simulink model "model_sinWave_1D"  (R2016b)
settings: Solver=FixedStepAuto  StartTime=0.0  StopTime=160  FixedStep=0.001  RelTol=1e-3  EnableMultiTasking=on
InitFcn:
  | initCallback_model1D
values from neighbouring files (symbols this model uses):
  f_sine = fArr(k)    [simulationMessung.m]
undefined symbols (not defined in the file or in its folder): C_phi, C_psi, g, I_GO, I_RM, l_AB, l_AC, m_K, m_R, phi_0, phi__d_0, phi_off, psi_0, psi__d_0, T_M_e, T_M_m
settings Model: Creator=ich  LastModifiedBy=ich
settings SolverCC: AutoInsertRateTranBlk=on
settings OptimizationCC: LifeSpan=inf
settings DebuggingCC: AlgebraicLoopMsg=none  SFUnexpectedBacktrackingDiag=warning  SFNoUnconditionalDefaultTransitionDiag=warning  SFExecutionAtInitializationDiag=none
settings GRTTargetCC: TargetLangStandard=C89/C90 (ANSI)  GeneratePreprocessorConditionals=Disable all
settings ConfigComp: CovMetricSettings=dw  CovHtmlReporting=on  CovSaveCumulativeToWorkspaceVar=on  CovSaveSingleToWorkspaceVar=on  CovExternalEMLEnable=off

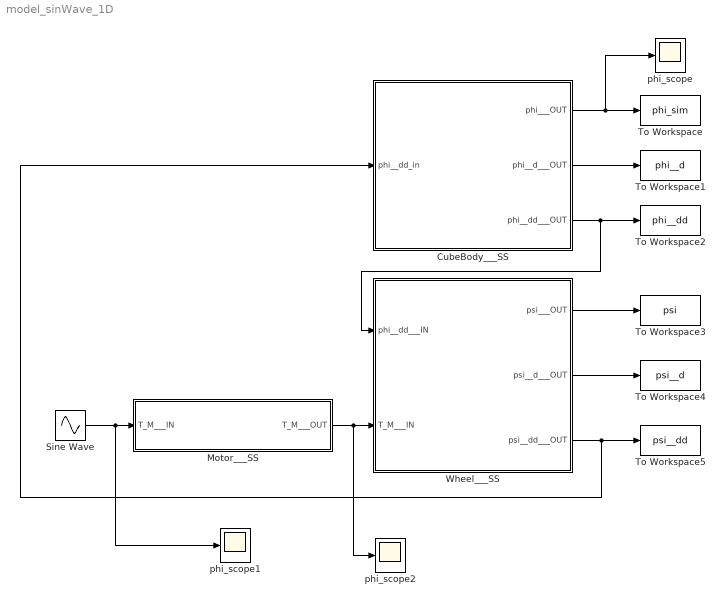
== system model_sinWave_1D ==
  CubeBody___SS : Subsystem
  Motor___SS : Subsystem
  Sine Wave : Sin  Amplitude=0.05  Frequency=2*pi*f_sine  SampleTime=0.02
  To Workspace : ToWorkspace  VariableName=phi_sim  SaveFormat=Timeseries  SampleTime=-1
  To Workspace1 : ToWorkspace  VariableName=phi__d  SaveFormat=Timeseries  SampleTime=-1
  To Workspace2 : ToWorkspace  VariableName=phi__dd  SaveFormat=Timeseries  SampleTime=-1
  To Workspace3 : ToWorkspace  VariableName=psi  SaveFormat=Timeseries  SampleTime=-1
  To Workspace4 : ToWorkspace  VariableName=psi__d  SaveFormat=Timeseries  SampleTime=-1
  To Workspace5 : ToWorkspace  VariableName=psi__dd  SaveFormat=Timeseries  SampleTime=-1
  Wheel___SS : Subsystem
  phi_scope : Scope
  phi_scope1 : Scope
  phi_scope2 : Scope
  wires:
  Motor___SS/1(T_M___OUT) -> phi_scope2/1, Wheel___SS/2(T_M___IN)
  CubeBody___SS/3(phi__dd___OUT) -> Wheel___SS/1(phi__dd___IN), To Workspace2/1
  Wheel___SS/3(psi__dd___OUT) -> To Workspace5/1, CubeBody___SS/1(phi__dd_in)
  CubeBody___SS/1(phi___OUT) -> phi_scope/1, To Workspace/1
  CubeBody___SS/2(phi__d___OUT) -> To Workspace1/1
  Wheel___SS/1(psi___OUT) -> To Workspace3/1
  Wheel___SS/2(psi__d___OUT) -> To Workspace4/1
  Sine Wave/1 -> phi_scope1/1, Motor___SS/1(T_M___IN)

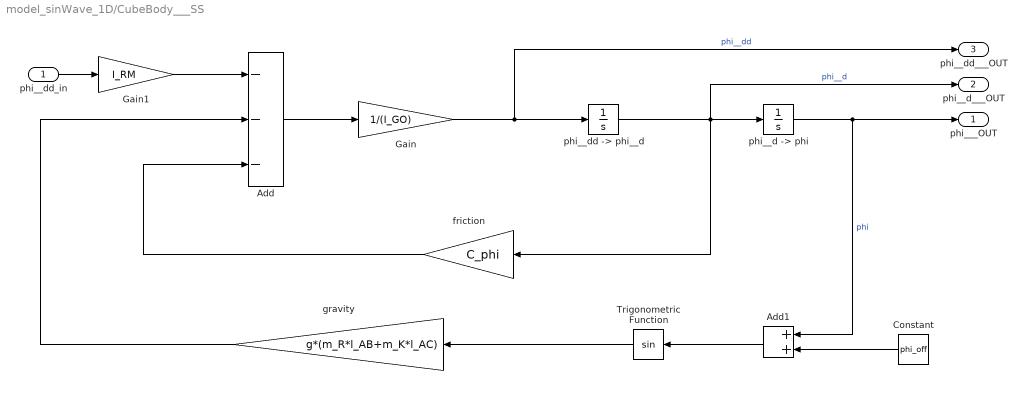
== system model_sinWave_1D/CubeBody___SS ==
  phi__dd_in : Inport
  Add : Sum  Inputs=---
  Add1 : Sum
  Constant : Constant  Value=phi_off
  Gain : Gain  Gain=1/(I_GO)
  Gain1 : Gain  Gain=I_RM
  Trigonometric Function : Trigonometry
  friction : Gain  Gain=C_phi
  gravity : Gain  Gain=g*(m_R*l_AB+m_K*l_AC)
  "phi__d -> phi" : Integrator  InitialCondition=phi_0
  "phi__dd -> phi__d" : Integrator  InitialCondition=phi__d_0
  phi___OUT : Outport
  phi__d___OUT : Outport  Port=2
  phi__dd___OUT : Outport  Port=3
  wires:
  "phi__d -> phi"/1 -> Add1/1, phi___OUT/1  "phi"
  "phi__dd -> phi__d"/1 -> friction/1, phi__d___OUT/1, "phi__d -> phi"/1  "phi__d"
  Gain/1 -> phi__dd___OUT/1, "phi__dd -> phi__d"/1  "phi__dd"
  Add/1 -> Gain/1
  phi__dd_in/1 -> Gain1/1
  Gain1/1 -> Add/1
  Trigonometric Function/1 -> gravity/1
  gravity/1 -> Add/2
  friction/1 -> Add/3
  Add1/1 -> Trigonometric Function/1
  Constant/1 -> Add1/2

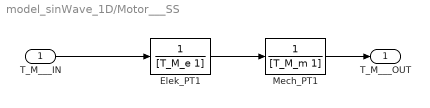
== system model_sinWave_1D/Motor___SS ==
  T_M___IN : Inport
  Elek_PT1 : TransferFcn  Denominator=[T_M_e 1]
  Mech_PT1 : TransferFcn  Denominator=[T_M_m 1]
  T_M___OUT : Outport
  wires:
  Elek_PT1/1 -> Mech_PT1/1
  Mech_PT1/1 -> T_M___OUT/1
  T_M___IN/1 -> Elek_PT1/1

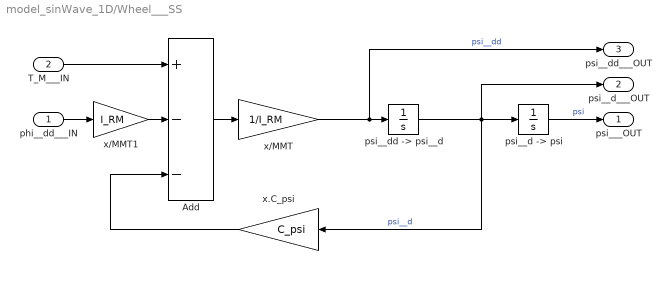
== system model_sinWave_1D/Wheel___SS ==
  phi__dd___IN : Inport
  T_M___IN : Inport  Port=2
  Add : Sum  Inputs=+--
  "psi__d -> psi" : Integrator  InitialCondition=psi_0
  "psi__dd -> psi__d" : Integrator  InitialCondition=psi__d_0
  x.C_psi : Gain  Gain=C_psi
  x/MMT : Gain  Gain=1/I_RM
  x/MMT1 : Gain  Gain=I_RM
  psi___OUT : Outport
  psi__d___OUT : Outport  Port=2
  psi__dd___OUT : Outport  Port=3
  wires:
  "psi__d -> psi"/1 -> psi___OUT/1  "psi"
  "psi__dd -> psi__d"/1 -> psi__d___OUT/1, "psi__d -> psi"/1, x.C_psi/1  "psi__d"
  x/MMT/1 -> psi__dd___OUT/1, "psi__dd -> psi__d"/1  "psi__dd"
  Add/1 -> x/MMT/1
  T_M___IN/1 -> Add/1
  x.C_psi/1 -> Add/3
  phi__dd___IN/1 -> x/MMT1/1
  x/MMT1/1 -> Add/2
